simulink library "TElib"  (Simulink 10.1)
settings: Solver=VariableStepAuto  StartTime=0.0  StopTime=10.0  RelTol=1e-3
undefined symbols (not defined in the file or in its folder): Ts
libraries: $bdroot x1
settings Model: Creator=s164106  LastModifiedBy=s164106

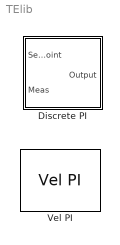
== system TElib ==
  Discrete PI : Subsystem  mask{Kc=0, Ti=inf, Ts=1, x0=0, Hi=1, Lo=-1}
  Vel PI : $bdroot/Discrete PI/Vel PI  Kc=Kc  Ti=Ti  Ts=Ts

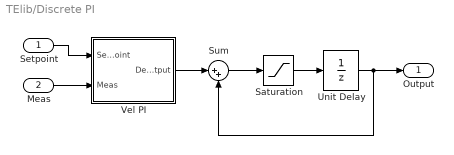
== system TElib/Discrete PI ==
  Setpoint : Inport
  Meas : Inport  Port=2
  Saturation : Saturate  UpperLimit=Hi  LowerLimit=Lo
  Sum : Sum  Inputs=|++  SaturateOnIntegerOverflow=on
  Unit Delay : UnitDelay  InitialCondition=x0  SampleTime=Ts
  Vel PI : Subsystem  mask{Kc=Kc, Ti=Ti, Ts=Ts}
  Output : Outport
  wires:
  Sum/1 -> Saturation/1
  Vel PI/1(Delta Output) -> Sum/1
  Saturation/1 -> Unit Delay/1
  Unit Delay/1 -> Sum/2, Output/1
  Meas/1 -> Vel PI/2(Meas)
  Setpoint/1 -> Vel PI/1(Setpoint)

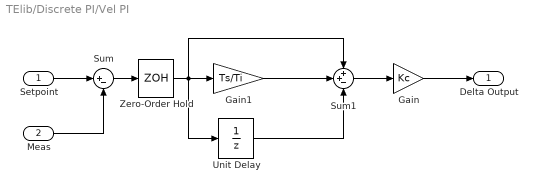
== system TElib/Discrete PI/Vel PI ==
  Setpoint : Inport
  Meas : Inport  Port=2
  Gain : Gain  Gain=Kc  SaturateOnIntegerOverflow=on  OutDataTypeStr=Inherit: Same as input  ParamDataTypeStr=Inherit: Same as input
  Gain1 : Gain  Gain=Ts/Ti  SaturateOnIntegerOverflow=on  OutDataTypeStr=Inherit: Same as input  ParamDataTypeStr=Inherit: Same as input
  Sum : Sum  Inputs=|+-  SaturateOnIntegerOverflow=on
  Sum1 : Sum  Inputs=++-  SaturateOnIntegerOverflow=on
  Unit Delay : UnitDelay  SampleTime=Ts
  Zero-Order Hold : ZeroOrderHold  SampleTime=Ts
  Delta Output : Outport
  wires:
  Setpoint/1 -> Sum/1
  Meas/1 -> Sum/2
  Gain/1 -> Delta Output/1
  Sum1/1 -> Gain/1
  Gain1/1 -> Sum1/2
  Unit Delay/1 -> Sum1/3
  Sum/1 -> Zero-Order Hold/1
  Zero-Order Hold/1 -> Gain1/1, Unit Delay/1, Sum1/1
